simulink model "zeroorderhold"  (Simulink 7.6)
settings: Solver=FixedStepDiscrete  StartTime=0.0  StopTime=10.0  FixedStep=1  RelTol=1e-3
settings Model: Creator=ksmyth  LastModifiedBy=hnine
settings OptimizationCC: InitFltsAndDblsToZero=on
settings DebuggingCC: SaveWithParameterizedLinksMsg=none  StrictBusMsg=Warning
settings GRTTargetCC: TargetFcnLib=ansi_tfl_tmw.mat

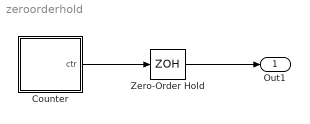
== system zeroorderhold ==
  Counter : Stateflow chart  TreatAsAtomicUnit=on
  Zero-Order Hold : ZeroOrderHold
  Out1 : Outport
  wires:
  Counter/1(ctr) -> Zero-Order Hold/1
  Zero-Order Hold/1 -> Out1/1

== stateflow chart Counter ==
  state s1
  (default) -> s1
  s1 -> s1 [order 1] : [ctr < 4] / ctr = ctr+1;
  s1 -> s1 [order 2] : [ctr >= 4] / ctr = -2;
  data: ctr output double =1
